simulink library "HardwareIO"  (R2014a)
settings: Solver=ode45  SolverMode=SingleTasking  StartTime=0.0  StopTime=10.0  RelTol=1e-3
values from neighbouring files (symbols this model uses):
  Ts = 0.002    [DSC_Control_Analysis.m]    (also in DSC_Control_Analysis_Exp.m; DSC_Speed_Control_Analysis.m; EC_params_nissan.m; Ext_MPCPara.m = SSD.Ts)
undefined symbols (not defined in the file or in its folder): bit, DiscIntNeverNeededParam, gr, Standard
libraries: canmsglib x6, xpcdiamondlib x2, simulink_extras x2, slrtsoftinglib x2, simulink x1
settings Model: Creator=Shad Laws  LastModifiedBy=cbeal

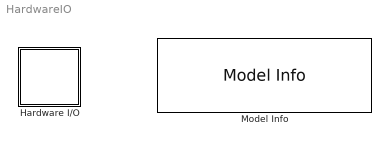
== system HardwareIO ==
  Hardware I/O : Subsystem
      mask init:
      | exist_p1_mdl = sum(strcmp(find_system('p1', 'searchdepth', 0), 'p1'));
      | 
      | if (exist_p1_mdl == 1)
      |     set_param('p1','StopTime','36000');
      |     set_param('p1','StartTime','0');
      | end
      mask Display: disp(['xPC\nI/O']);
  Model Info : simulink/Model-Wide Utilities/Model Info  InitialBlockCM=None  BlockCM=none  Frame=off  DisplayStringWithTags=|  HorizontalTextAlignment=Left  LeftAlignmentValue=0.02  SourceBlockDiagram=HardwareIO  TagMaxNumber=20
      | Last saved on: %<LastModificationDate>
      | Save number: %<ModelVersion>
      | $Revision: 647 $
      | $URL: https://nissan.stanford.edu/nissanxpc/development/HardwareIO.mdl $

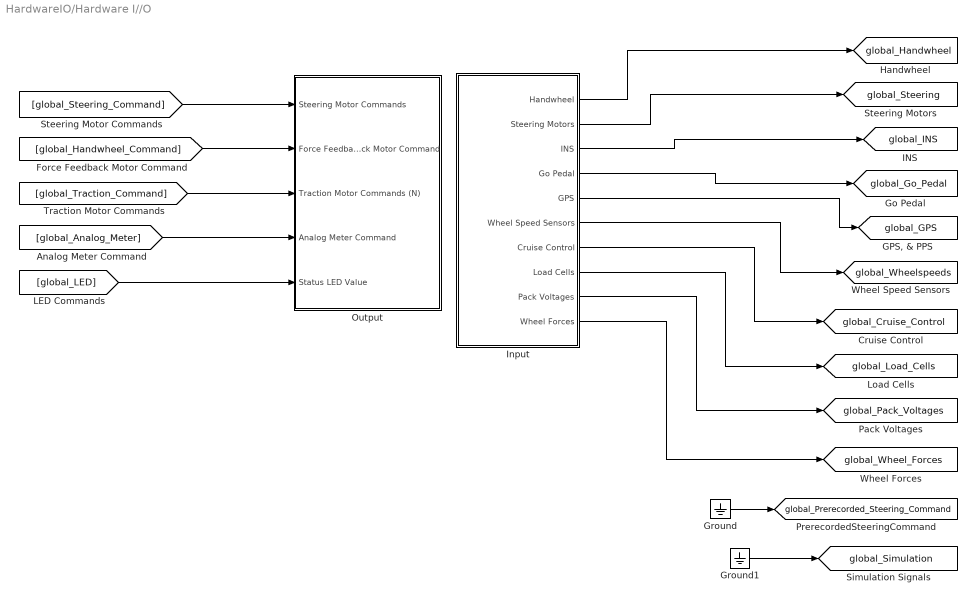
== system HardwareIO/Hardware I//O ==
  Ground : Ground
  Ground1 : Ground
  Input : Subsystem
  Output : Subsystem
  tag scope: global_Cruise_Control=global, global_GPS=global, global_Go_Pedal=global, global_Handwheel=global, global_INS=global, global_Load_Cells=global, global_Pack_Voltages=global, global_Prerecorded_Steering_Command=global, global_Simulation=global, global_Steering=global, global_Wheel_Forces=global, global_Wheelspeeds=global
  wires:
  Input/10(Wheel Forces) -> [global_Wheel_Forces]
  Input/9(Pack Voltages) -> [global_Pack_Voltages]
  Input/8(Load Cells) -> [global_Load_Cells]
  [global_Traction_Command] -> Output/3(Traction Motor Commands (N))
  [global_Analog_Meter] -> Output/4(Analog Meter Command)
  [global_Steering_Command] -> Output/1(Steering Motor Commands)
  [global_Handwheel_Command] -> Output/2(Force Feedback Motor Command)
  [global_LED] -> Output/5(Status LED Value)
  Input/1(Handwheel) -> [global_Handwheel]
  Input/2(Steering Motors) -> [global_Steering]
  Input/3(INS) -> [global_INS]
  Input/4(Go Pedal) -> [global_Go_Pedal]
  Input/5(GPS) -> [global_GPS]
  Input/6(Wheel Speed Sensors) -> [global_Wheelspeeds]
  Input/7(Cruise Control) -> [global_Cruise_Control]
  Ground/1 -> [global_Prerecorded_Steering_Command]
  Ground1/1 -> [global_Simulation]

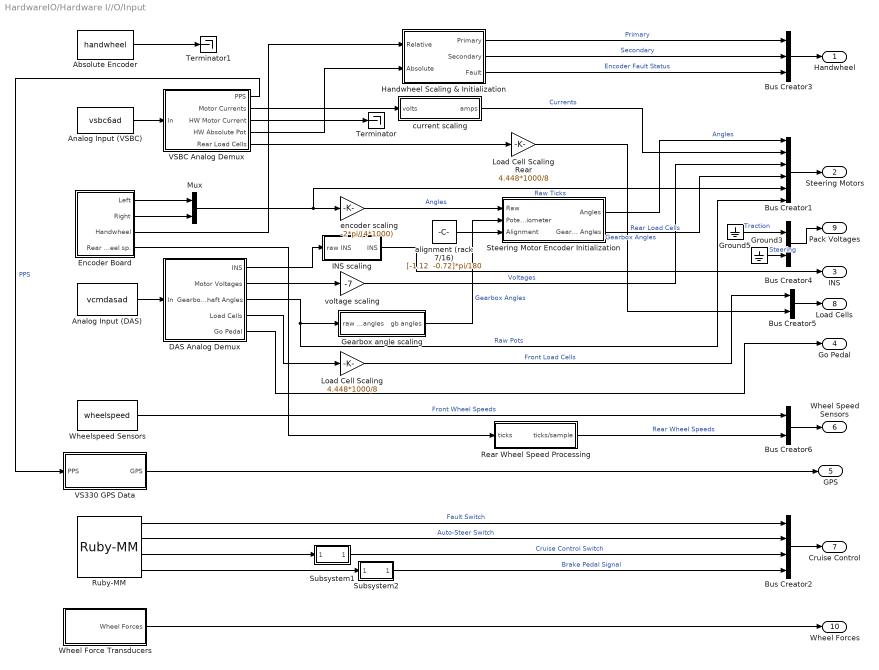
== system HardwareIO/Hardware I//O/Input ==
  Absolute Encoder : S-Function  FunctionName=handwheel  Parameters=Ts  EnableBusSupport=off
  Analog Input (DAS) : S-Function  FunctionName=vcmdasad  Parameters=numChannels, inputVec, sampleTime  EnableBusSupport=off  mask{numChannels=16, inputVec=[4 4 4 4 4 4 4 4 4 4 4 4 4 4 4 4], sampleTime=Ts}
      mask prompts: sampleTime "sample_time"
  Analog Input (VSBC) : S-Function  FunctionName=vsbc6ad  Parameters=numChannels,inpRange,sampTime  EnableBusSupport=off  mask{numChannels=8, inpRange=[4 4 1 4 4 3 3 2], sampTime=Ts}
      mask prompts: numChannels "Number of Channels"; inpRange "Analog Input Range (1: +5; 2: +10; 3: +-5; 4: +-10)"; sampTime "Sampling Time"
  Bus Creator1 : BusCreator  Inputs=6
  Bus Creator2 : BusCreator
  Bus Creator3 : BusCreator  Inputs=3
  Bus Creator4 : BusCreator  Inputs=2
  Bus Creator5 : BusCreator  Inputs=2
  Bus Creator6 : BusCreator  Inputs=2
  DAS Analog Demux : Subsystem
  Encoder Board : Subsystem
  Gearbox angle scaling : Subsystem
  Ground3 : Ground
  Ground5 : Ground
  Handwheel Scaling & Initialization : Subsystem
  INS scaling : Subsystem
  Load Cell Scaling : Gain  Gain=4.448*1000/8  SaturateOnIntegerOverflow=on  OutDataTypeStr=Inherit: Same as input  ParamDataTypeStr=Inherit: Same as input
  Load Cell Scaling Rear : Gain  Gain=4.448*1000/8  SaturateOnIntegerOverflow=on  OutDataTypeStr=Inherit: Same as input  ParamDataTypeStr=Inherit: Same as input
  Mux : Mux  Inputs=2
  Rear Wheel Speed Processing : Subsystem
  Ruby-MM : xpcdiamondlib/Digital Input/Ruby-MM   channel=[5 6 7 8]  port=A  chip=1  sampletime=Ts  baseaddress=0x300
  Steering Motor Encoder Initialization : Subsystem
      mask init:
      | p1_params
  Subsystem1 : Subsystem
      mask Display: disp('!');
  Subsystem2 : Subsystem
      mask Display: disp('!');
  Terminator : Terminator
  Terminator1 : Terminator
  VS330 GPS Data : Subsystem
  VSBC Analog Demux : Subsystem
  Wheel Force Transducers : Subsystem
  Wheelspeed Sensors : S-Function  FunctionName=wheelspeed  Parameters=Ts  EnableBusSupport=off
  alignment (rack 7/16) : Constant  Value="[-1.12  -0.72]*pi/180"
  current scaling : Subsystem
  encoder scaling : Gain  Gain=-2*pi/(4*1000)  SaturateOnIntegerOverflow=on  OutDataTypeStr=Inherit: Same as input  ParamDataTypeStr=Inherit: Same as input
  voltage scaling : Gain  Gain=-7  SaturateOnIntegerOverflow=on  OutDataTypeStr=Inherit: Same as input  ParamDataTypeStr=Inherit: Same as input
  Handwheel : Outport
  Steering Motors : Outport  Port=2
  INS : Outport  Port=3
  Go Pedal : Outport  Port=4
  GPS : Outport  Port=5
  Wheel Speed Sensors : Outport  Port=6
  Cruise Control : Outport  Port=7
  Load Cells : Outport  Port=8
  Pack Voltages : Outport  Port=9
  Wheel Forces : Outport  Port=10
  wires:
  VS330 GPS Data/1(GPS) -> GPS/1
  Wheel Force Transducers/1(Wheel Forces) -> Wheel Forces/1
  Bus Creator6/1 -> Wheel Speed Sensors/1
  Encoder Board/4(Rear wheel sp.) -> Rear Wheel Speed Processing/1(ticks)
  Rear Wheel Speed Processing/1(ticks/sample) -> Bus Creator6/2  "Rear Wheel Speeds"
  Wheelspeed Sensors/1 -> Bus Creator6/1  "Front Wheel Speeds"
  Bus Creator5/1 -> Load Cells/1
  Load Cell Scaling Rear/1 -> Bus Creator5/2  "Rear Load Cells"
  VSBC Analog Demux/5(Rear Load Cells) -> Load Cell Scaling Rear/1
  Load Cell Scaling/1 -> Bus Creator5/1  "Front Load Cells"
  Absolute Encoder/1 -> Terminator1/1
  VSBC Analog Demux/3(HW Motor Current) -> Terminator/1
  Encoder Board/3(Handwheel) -> Handwheel Scaling & Initialization/1(Relative)
  Ground3/1 -> Bus Creator4/2  "Steering"
  Bus Creator4/1 -> Pack Voltages/1
  DAS Analog Demux/4(Load Cells) -> Load Cell Scaling/1
  Handwheel Scaling & Initialization/2(Secondary) -> Bus Creator3/2  "Secondary"
  Bus Creator3/1 -> Handwheel/1
  DAS Analog Demux/5(Go Pedal) -> Go Pedal/1
  Bus Creator2/1 -> Cruise Control/1
  DAS Analog Demux/2(Motor Voltages) -> voltage scaling/1
  voltage scaling/1 -> Bus Creator1/3  "Voltages"
  Mux/1 -> encoder scaling/1, Bus Creator1/5  "Raw Ticks"
  Encoder Board/2(Right) -> Mux/2
  Encoder Board/1(Left) -> Mux/1
  Analog Input (VSBC)/1 -> VSBC Analog Demux/1(In)
  VSBC Analog Demux/1(PPS) -> VS330 GPS Data/1(PPS)  "PPS"
  Bus Creator1/1 -> Steering Motors/1
  VSBC Analog Demux/2(Motor Currents) -> current scaling/1(volts)
  current scaling/1(amps) -> Bus Creator1/2  "Currents"
  INS scaling/1(INS) -> INS/1
  DAS Analog Demux/1(INS) -> INS scaling/1(raw INS)
  Analog Input (DAS)/1 -> DAS Analog Demux/1(In)
  DAS Analog Demux/3(Gearbox Shaft Angles) -> Bus Creator1/6, Gearbox angle scaling/1(raw gb angles)  "Raw Pots"
  Gearbox angle scaling/1(gb angles) -> Steering Motor Encoder Initialization/2(Potentiometer)  "Gearbox Angles"
  Subsystem1/1(Out1) -> Bus Creator2/3  "Cruise Control Switch"
  Subsystem2/1(Out1) -> Bus Creator2/4  "Brake Pedal Signal"
  encoder scaling/1 -> Steering Motor Encoder Initialization/1(Raw)  "Angles"
  Handwheel Scaling & Initialization/3(Fault) -> Bus Creator3/3  "Encoder Fault Status"
  Steering Motor Encoder Initialization/1(Angles) -> Bus Creator1/1  "Angles"
  alignment (rack 7/16)/1 -> Steering Motor Encoder Initialization/3(Alignment)
  Steering Motor Encoder Initialization/2(Gearbox Angles) -> Bus Creator1/4  "Gearbox Angles"
  Ruby-MM/3 -> Subsystem1/1(In1)
  Ruby-MM/4 -> Subsystem2/1(In1)
  Ruby-MM/2 -> Bus Creator2/2  "Auto-Steer Switch"
  Ruby-MM/1 -> Bus Creator2/1  "Fault Switch"
  Ground5/1 -> Bus Creator4/1  "Traction"
  Handwheel Scaling & Initialization/1(Primary) -> Bus Creator3/1  "Primary"
  VSBC Analog Demux/4(HW Absolute Pot) -> Handwheel Scaling & Initialization/2(Absolute)

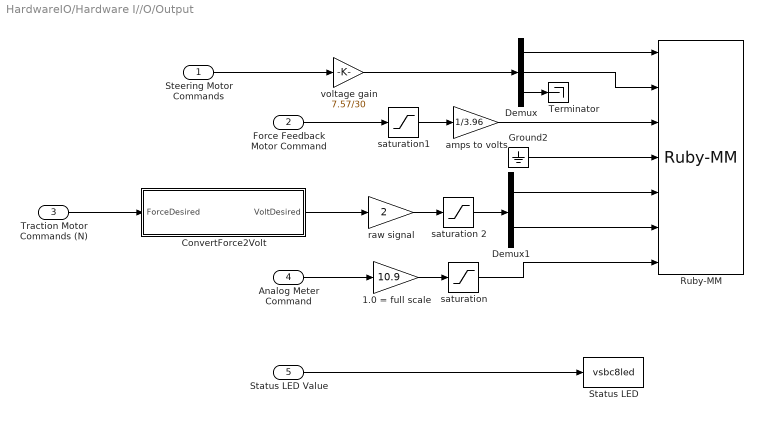
== system HardwareIO/Hardware I//O/Output ==
  Steering Motor Commands : Inport
  Force Feedback Motor Command : Inport  Port=2
  Traction Motor Commands (N) : Inport  Port=3
  Analog Meter Command : Inport  Port=4
  Status LED Value : Inport  Port=5
  1.0 = full scale : Gain  Gain=10.9  SaturateOnIntegerOverflow=on  OutDataTypeStr=Inherit: Same as input  ParamDataTypeStr=Inherit: Same as input
  ConvertForce2Volt : Subsystem  TreatAsAtomicUnit=on
  Demux : Demux  Outputs=[1 1 -1]
  Demux1 : Demux  Outputs=2
  Ground2 : Ground
  "Ruby-MM " : xpcdiamondlib/D//A/Ruby-MM   channel=[1 2 3 4 5 6 7]  range0=+-10  range1=+-10  reset=[1 1 1 1 1 1 1]  initValue=[0 0 0 0 0 0 0]  st=Ts  baseaddress=0x300
  Status LED : S-Function  FunctionName=vsbc8led  EnableBusSupport=off
  Terminator : Terminator
  amps to volts : Gain  Gain=1/3.96  SaturateOnIntegerOverflow=on  OutDataTypeStr=Inherit: Same as input  ParamDataTypeStr=Inherit: Same as input
  raw signal : Gain  Gain=2  SaturateOnIntegerOverflow=on  OutDataTypeStr=Inherit: Same as input  ParamDataTypeStr=Inherit: Same as input
  saturation : Saturate  UpperLimit=11  LowerLimit=0
  saturation 2 : Saturate  UpperLimit=6  LowerLimit=0  OutDataTypeStr=Inherit: Inherit via back propagation
  saturation1 : Saturate  UpperLimit=2  LowerLimit=-2
  voltage gain : Gain  Gain=7.57/30  SaturateOnIntegerOverflow=on  OutDataTypeStr=Inherit: Same as input  ParamDataTypeStr=Inherit: Same as input
  wires:
  Demux/3 -> Terminator/1
  ConvertForce2Volt/1(VoltDesired) -> raw signal/1
  amps to volts/1 -> "Ruby-MM "/3
  Force Feedback Motor Command/1 -> saturation1/1
  raw signal/1 -> saturation 2/1
  saturation 2/1 -> Demux1/1
  saturation/1 -> "Ruby-MM "/7
  Demux1/2 -> "Ruby-MM "/6
  Steering Motor Commands/1 -> voltage gain/1
  voltage gain/1 -> Demux/1
  1.0 = full scale/1 -> saturation/1
  Ground2/1 -> "Ruby-MM "/4
  Demux/2 -> "Ruby-MM "/2
  Demux/1 -> "Ruby-MM "/1
  Status LED Value/1 -> Status LED/1
  Demux1/1 -> "Ruby-MM "/5
  Traction Motor Commands (N)/1 -> ConvertForce2Volt/1(ForceDesired)
  Analog Meter Command/1 -> 1.0 = full scale/1
  saturation1/1 -> amps to volts/1

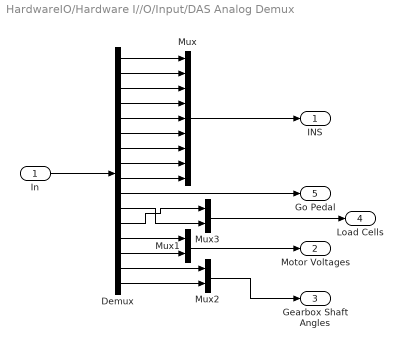
== system HardwareIO/Hardware I//O/Input/DAS Analog Demux ==
  In : Inport
  Demux : Demux  Outputs=16
  Mux : Mux  Inputs=9
  Mux1 : Mux  Inputs=2
  Mux2 : Mux  Inputs=2
  Mux3 : Mux  Inputs=2
  INS : Outport
  Motor Voltages : Outport  Port=2
  Gearbox Shaft Angles : Outport  Port=3
  Load Cells : Outport  Port=4
  Go Pedal : Outport  Port=5
  wires:
  Demux/10 -> Go Pedal/1
  Mux3/1 -> Load Cells/1
  Demux/16 -> Mux2/2
  Demux/15 -> Mux2/1
  Demux/2 -> Mux/2
  Demux/14 -> Mux1/2
  Demux/13 -> Mux1/1
  Mux1/1 -> Motor Voltages/1
  Mux/1 -> INS/1
  Demux/9 -> Mux/9
  Demux/8 -> Mux/8
  Demux/7 -> Mux/7
  Demux/6 -> Mux/6
  Demux/5 -> Mux/5
  Demux/4 -> Mux/4
  Demux/3 -> Mux/3
  Demux/1 -> Mux/1
  In/1 -> Demux/1
  Mux2/1 -> Gearbox Shaft Angles/1
  Demux/11 -> Mux3/2
  Demux/12 -> Mux3/1

== system HardwareIO/Hardware I//O/Input/Encoder Board ==
  Mux : Mux  Inputs=2
  "encoder board " : S-Function  FunctionName=UltimateEncoder  Parameters=TSamp,NC,BA,[R1 R2 R3 R4 R5 R6 ]  EnableBusSupport=off  mask{TSamp=Ts, BA=528, NC=5, R1=on, R2=on, R3=on, R4=off, R5=off, R6=off}
      mask prompts: TSamp "Sampling Rate"; BA "Base Adress (Base 10)"; NC "Number of Channels"; R1 "Unwrap Channel 1"; R2 "Unwrap Channel 2"; R3 "Unwrap Channel 3"; R4 "Unwrap Channel 4"; R5 "Unwrap Channel 5"; R6 "Unwrap Channel 6"
  reset : Constant  Value=[1 1 1 0 0]
  Left : Outport
  Right : Outport  Port=2
  Handwheel : Outport  Port=3
  Rear wheel sp. : Outport  Port=4
  wires:
  Mux/1 -> Rear wheel sp./1
  "encoder board "/5 -> Mux/2
  "encoder board "/4 -> Mux/1
  "encoder board "/3 -> Handwheel/1
  reset/1 -> "encoder board "/1
  "encoder board "/1 -> Left/1
  "encoder board "/2 -> Right/1

== system HardwareIO/Hardware I//O/Input/Gearbox angle scaling ==
  raw gb angles : Inport
  Pot readings with wheels centered : Constant  Value=[ -2.041; -1.733 ]
  Sum : Sum  Inputs=|++  SaturateOnIntegerOverflow=on
  Volts/Rad (Left/right pots wired in reverse) : Gain  Gain=[1/ -1.31; 1/1.254]  SaturateOnIntegerOverflow=on  OutDataTypeStr=Inherit: Same as input  ParamDataTypeStr=Inherit: Same as input
  gb angles : Outport
  wires:
  Sum/1 -> Volts/Rad (Left/right pots wired in reverse)/1
  raw gb angles/1 -> Sum/1
  Pot readings with wheels centered/1 -> Sum/2
  Volts/Rad (Left/right pots wired in reverse)/1 -> gb angles/1

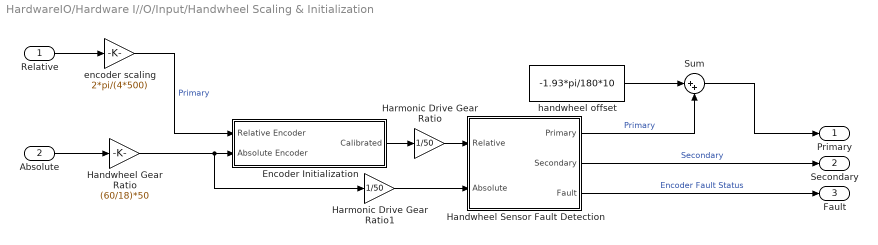
== system HardwareIO/Hardware I//O/Input/Handwheel Scaling & Initialization ==
  Relative : Inport
  Absolute : Inport  Port=2
  Encoder Initialization : Subsystem
  Handwheel Gear Ratio : Gain  Gain=(60/18)*50  SaturateOnIntegerOverflow=on  OutDataTypeStr=Inherit: Same as input  ParamDataTypeStr=Inherit: Same as input
  Handwheel Sensor Fault Detection : Subsystem
  Harmonic Drive Gear Ratio : Gain  Gain=1/50  SaturateOnIntegerOverflow=on  OutDataTypeStr=Inherit: Same as input  ParamDataTypeStr=Inherit: Same as input
  Harmonic Drive Gear Ratio1 : Gain  Gain=1/50  SaturateOnIntegerOverflow=on  OutDataTypeStr=Inherit: Same as input  ParamDataTypeStr=Inherit: Same as input
  Sum : Sum  Inputs=|++
  encoder scaling : Gain  Gain=2*pi/(4*500)  SaturateOnIntegerOverflow=on  OutDataTypeStr=Inherit: Same as input  ParamDataTypeStr=Inherit: Same as input
  handwheel offset : Constant  Value=-1.93*pi/180*10
  Primary : Outport
  Secondary : Outport  Port=2
  Fault : Outport  Port=3
  wires:
  Handwheel Sensor Fault Detection/1(Primary) -> Sum/2  "Primary"
  Sum/1 -> Primary/1
  handwheel offset/1 -> Sum/1
  Harmonic Drive Gear Ratio1/1 -> Handwheel Sensor Fault Detection/2(Absolute)
  Absolute/1 -> Handwheel Gear Ratio/1
  Relative/1 -> encoder scaling/1
  Harmonic Drive Gear Ratio/1 -> Handwheel Sensor Fault Detection/1(Relative)
  Handwheel Sensor Fault Detection/2(Secondary) -> Secondary/1  "Secondary"
  Encoder Initialization/1(Calibrated) -> Harmonic Drive Gear Ratio/1
  Handwheel Sensor Fault Detection/3(Fault) -> Fault/1  "Encoder Fault Status"
  Handwheel Gear Ratio/1 -> Harmonic Drive Gear Ratio1/1, Encoder Initialization/2(Absolute Encoder)
  encoder scaling/1 -> Encoder Initialization/1(Relative Encoder)  "Primary"

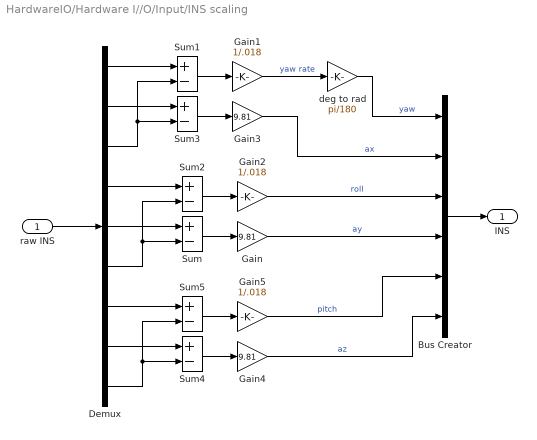
== system HardwareIO/Hardware I//O/Input/INS scaling ==
  raw INS : Inport
  Bus Creator : BusCreator  Inputs=6
  Demux : Demux  Outputs=9
  Gain : Gain  Gain=9.81  SaturateOnIntegerOverflow=on  OutDataTypeStr=Inherit: Same as input  ParamDataTypeStr=Inherit: Same as input
  Gain1 : Gain  Gain=1/.018  SaturateOnIntegerOverflow=on  OutDataTypeStr=Inherit: Same as input  ParamDataTypeStr=Inherit: Same as input
  Gain2 : Gain  Gain=1/.018  SaturateOnIntegerOverflow=on  OutDataTypeStr=Inherit: Same as input  ParamDataTypeStr=Inherit: Same as input
  Gain3 : Gain  Gain=9.81  SaturateOnIntegerOverflow=on  OutDataTypeStr=Inherit: Same as input  ParamDataTypeStr=Inherit: Same as input
  Gain4 : Gain  Gain=9.81  SaturateOnIntegerOverflow=on  OutDataTypeStr=Inherit: Same as input  ParamDataTypeStr=Inherit: Same as input
  Gain5 : Gain  Gain=1/.018  SaturateOnIntegerOverflow=on  OutDataTypeStr=Inherit: Same as input  ParamDataTypeStr=Inherit: Same as input
  Sum{,1..5} (6 alike) : Sum  Inputs=+-  SaturateOnIntegerOverflow=on  InputSameDT=on  OutDataTypeStr=Inherit: Same as first input
  deg to rad : Gain  Gain=pi/180  SaturateOnIntegerOverflow=on  OutDataTypeStr=Inherit: Same as input  ParamDataTypeStr=Inherit: Same as input
  INS : Outport
  wires:
  Bus Creator/1 -> INS/1
  deg to rad/1 -> Bus Creator/1  "yaw"
  Demux/9 -> Sum4/2, Sum5/2
  Demux/5 -> Sum/1
  Demux/8 -> Sum4/1
  Demux/7 -> Sum5/1
  Sum4/1 -> Gain4/1
  Sum5/1 -> Gain5/1
  Gain4/1 -> Bus Creator/6  "az"
  Gain5/1 -> Bus Creator/5  "pitch"
  raw INS/1 -> Demux/1
  Sum/1 -> Gain/1
  Sum1/1 -> Gain1/1
  Sum2/1 -> Gain2/1
  Sum3/1 -> Gain3/1
  Gain/1 -> Bus Creator/4  "ay"
  Gain1/1 -> deg to rad/1  "yaw rate"
  Gain2/1 -> Bus Creator/3  "roll"
  Gain3/1 -> Bus Creator/2  "ax"
  Demux/1 -> Sum1/1
  Demux/3 -> Sum1/2, Sum3/2
  Demux/2 -> Sum3/1
  Demux/4 -> Sum2/1
  Demux/6 -> Sum/2, Sum2/2

== system HardwareIO/Hardware I//O/Input/Rear Wheel Speed Processing ==
  ticks : Inport
  Demux : Demux  Outputs=2
  Mux : Mux  Inputs=2
  Speed Calc : Subsystem  mask{range=65536}
      mask prompts: range "Wrap range"
      mask Display: disp(range);
  Speed Calc1 : Subsystem  mask{range=65536}
      mask prompts: range "Wrap range"
      mask Display: disp(range);
  de-quadrature : Gain  Gain=1/2
  ticks/sample : Outport
  wires:
  de-quadrature/1 -> ticks/sample/1
  Mux/1 -> de-quadrature/1
  Speed Calc1/1(Speed) -> Mux/2
  Demux/2 -> Speed Calc1/1(Distance)
  Speed Calc/1(Speed) -> Mux/1
  Demux/1 -> Speed Calc/1(Distance)
  ticks/1 -> Demux/1

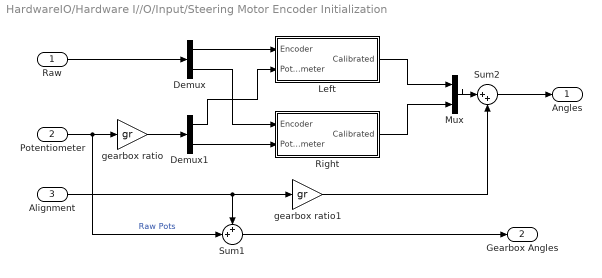
== system HardwareIO/Hardware I//O/Input/Steering Motor Encoder Initialization ==
  Raw : Inport
  Potentiometer : Inport  Port=2
  Alignment : Inport  Port=3
  Demux : Demux  Outputs=2
  Demux1 : Demux  Outputs=2
  Left : Subsystem
  Mux : Mux  Inputs=2
  Right : Subsystem
  Sum1 : Sum  Inputs=++|
  Sum2 : Sum  Inputs=|++
  gearbox ratio : Gain  Gain=gr  SaturateOnIntegerOverflow=on  OutDataTypeStr=Inherit: Same as input  ParamDataTypeStr=Inherit: Same as input
  gearbox ratio1 : Gain  Gain=gr  SaturateOnIntegerOverflow=on  OutDataTypeStr=Inherit: Same as input  ParamDataTypeStr=Inherit: Same as input
  Angles : Outport
  Gearbox Angles : Outport  Port=2
  wires:
  Demux1/2 -> Right/2(Potentiometer)
  Demux1/1 -> Left/2(Potentiometer)
  Demux/2 -> Right/1(Encoder)
  Demux/1 -> Left/1(Encoder)
  Left/1(Calibrated) -> Mux/1
  Potentiometer/1 -> gearbox ratio/1, Sum1/2  "Raw Pots"
  Raw/1 -> Demux/1
  gearbox ratio/1 -> Demux1/1
  Right/1(Calibrated) -> Mux/2
  Mux/1 -> Sum2/1
  Sum2/1 -> Angles/1
  Alignment/1 -> gearbox ratio1/1, Sum1/1
  gearbox ratio1/1 -> Sum2/2
  Sum1/1 -> Gearbox Angles/1

== system HardwareIO/Hardware I//O/Input/Subsystem1 ==
  In1 : Inport
  Constant : Constant
  Sum : Sum  Inputs=+-|
  Out1 : Outport
  wires:
  Constant/1 -> Sum/1
  In1/1 -> Sum/2
  Sum/1 -> Out1/1

== system HardwareIO/Hardware I//O/Input/Subsystem2 ==
  In1 : Inport
  Constant : Constant
  Sum : Sum  Inputs=+-|
  Out1 : Outport
  wires:
  Sum/1 -> Out1/1
  In1/1 -> Sum/2
  Constant/1 -> Sum/1

== system HardwareIO/Hardware I//O/Input/VS330 GPS Data ==
  note: Do not reorder the signals in
      | GPS or DataDescription will
      | not match the data.
  PPS : Inport
  Bus Creator : BusCreator  Inputs=28
  Demux : Demux  Outputs=24
  Hemisphere VS330 : S-Function  FunctionName=vs330_bin3_rcv  Parameters=Ts  EnableBusSupport=off
  Roll Axis Reversed : Gain  Gain=-1
  Subsystem : Subsystem
  Terminator2 : Terminator
  GPS : Outport
  wires:
  Roll Axis Reversed/1 -> Bus Creator/14  "Roll Angle"
  Demux/12 -> Roll Axis Reversed/1  "Roll Angle"
  Subsystem/3(Z) -> Bus Creator/9  "ECEF Z"
  Subsystem/2(Y) -> Bus Creator/8  "ECEF Y"
  Subsystem/1(X) -> Bus Creator/7  "ECEF X"
  Demux/7 -> Bus Creator/6, Subsystem/3(Alt)  "Altitude"
  Demux/6 -> Bus Creator/5, Subsystem/2(Long)  "Longitude"
  Demux/5 -> Bus Creator/4, Subsystem/1(Lat)  "Latitude"
  Demux/18 -> Bus Creator/22  "Vert RMS"
  Demux/23 -> Bus Creator/27  "Cov EU"
  Demux/14 -> Bus Creator/16  "Attitude Status"
  Demux/15 -> Bus Creator/19  "Yaw stddev"
  Demux/21 -> Bus Creator/25  "Cov NU"
  Demux/1 -> Bus Creator/2  "ToW"
  Demux/17 -> Bus Creator/21  "Hor RMS"
  Demux/4 -> Bus Creator/15  "Nav Mode"
  Demux/3 -> Bus Creator/17  "Sats Used"
  Demux/22 -> Bus Creator/26  "Cov EE"
  Demux/20 -> Bus Creator/24  "Cov NE"
  Demux/24 -> Bus Creator/28  "Cov UU"
  Demux/11 -> Bus Creator/13  "Heading"
  Demux/2 -> Bus Creator/3  "Wk Num"
  Demux/19 -> Bus Creator/23  "Cov NN"
  Demux/9 -> Bus Creator/11  "Vert Vel"
  Demux/8 -> Bus Creator/10  "Hor Speed"
  Demux/10 -> Bus Creator/12  "CoG"
  Demux/13 -> Bus Creator/18  "Diff Age"
  Demux/16 -> Bus Creator/20  "Roll stddev"
  Hemisphere VS330/1 -> Demux/1
  Hemisphere VS330/2 -> Terminator2/1
  Bus Creator/1 -> GPS/1
  PPS/1 -> Bus Creator/1

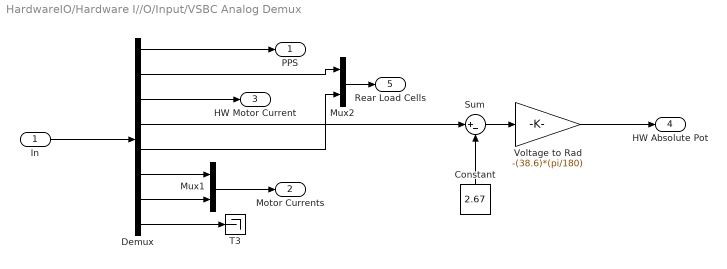
== system HardwareIO/Hardware I//O/Input/VSBC Analog Demux ==
  In : Inport
  Constant : Constant  Value=2.67
  Demux : Demux  Outputs=8
  Mux1 : Mux  Inputs=2
  Mux2 : Mux  Inputs=2
  Sum : Sum  Inputs=|+-
  T3 : Terminator
  Voltage to Rad : Gain  Gain=-(38.6)*(pi/180)
  PPS : Outport
  Motor Currents : Outport  Port=2
  HW Motor Current : Outport  Port=3
  HW Absolute Pot : Outport  Port=4
  Rear Load Cells : Outport  Port=5
  wires:
  Mux2/1 -> Rear Load Cells/1
  Demux/5 -> Mux2/2
  Demux/2 -> Mux2/1
  Constant/1 -> Sum/2
  Sum/1 -> Voltage to Rad/1
  Demux/4 -> Sum/1
  Voltage to Rad/1 -> HW Absolute Pot/1
  Demux/8 -> T3/1
  Demux/1 -> PPS/1
  Demux/3 -> HW Motor Current/1
  Demux/6 -> Mux1/1
  Demux/7 -> Mux1/2
  In/1 -> Demux/1
  Mux1/1 -> Motor Currents/1

== system HardwareIO/Hardware I//O/Input/Wheel Force Transducers ==
  Bus Creator : BusCreator  Inputs=20
  CAN Unpack : canmsglib/CAN Unpack  MsgList=(none)  MsgName=CAN Msg  MsgIDType=Standard (11-bit identifier)  MsgIdentifier=460  MsgLength=8  SignalInfo=LF_X_Force$0$16$1$1$1$0$1.220703125$0$-Inf$Inf$#LF_Y_Force$16$16$1$1$1$0$0.6103515625$0$-Inf$Inf$#LF_Z_Force$32$16$1$1$1$0$1.220703125$0$-Inf$Inf$#LF_MX_Moment$48$16$1$1$1$0$0.18310546875$0$-Inf$Inf$#  NSignals=4  IDPort=off  TimestampPort=off  ErrorPort=off  RemotePort=off  LengthPort=off  StatusPort=on  StartBits=str2num('[int32(0);int32(16);int32(32);int32(48)]')  SignalSizes=str2num('[int32(16);int32(16);int32(16);int32(16)]')  ByteOrders=str2num('[int32(1);int32(1);int32(1);int32(1)]')  DataTypes=str2num('[int32(1);int32(1);int32(1);int32(1)]')  MultiplexTypes=str2num('[int32(1);int32(1);int32(1);int32(1)]')  MultiplexValues=str2num('[double(0);double(0);double(0);double(0)]')  Factors=str2num('[double(1.220703125);double(0.6103515625);double(1.220703125);double(0.18310546875)]')  Offsets=str2num('[double(0);double(0);double(0);double(0)]')  Minimums=str2num('[double(-Inf);double(-Inf);double(-Inf);double(-Inf)]')  Maximums=str2num('[double(Inf);double(Inf);double(Inf);double(Inf)]')
  CAN Unpack1 : canmsglib/CAN Unpack  MsgList=(none)  MsgName=CAN Msg  MsgIDType=Standard (11-bit identifier)  MsgIdentifier=1484  MsgLength=8  SignalInfo=LF_MY_Moment$0$16$1$1$1$0$0.18310546875$0$-Inf$Inf$#LF_MZ_Moment$16$16$1$1$1$0$0.18310546875$0$-Inf$Inf$#LF_Velocity$32$16$1$1$1$0$0.06103515625$0$-Inf$Inf$#LF_Position$48$16$1$1$1$0$0.010986328125$0$-Inf$Inf$#  NSignals=4  IDPort=off  TimestampPort=off  ErrorPort=off  RemotePort=off  LengthPort=off  StatusPort=on  StartBits=str2num('[int32(0);int32(16);int32(32);int32(48)]')  SignalSizes=str2num('[int32(16);int32(16);int32(16);int32(16)]')  ByteOrders=str2num('[int32(1);int32(1);int32(1);int32(1)]')  DataTypes=str2num('[int32(1);int32(1);int32(1);int32(1)]')  MultiplexTypes=str2num('[int32(1);int32(1);int32(1);int32(1)]')  MultiplexValues=str2num('[double(0);double(0);double(0);double(0)]')  Factors=str2num('[double(0.18310546875);double(0.18310546875);double(0.06103515625);double(0.010986328125)]')  Offsets=str2num('[double(0);double(0);double(0);double(0)]')  Minimums=str2num('[double(-Inf);double(-Inf);double(-Inf);double(-Inf)]')  Maximums=str2num('[double(Inf);double(Inf);double(Inf);double(Inf)]')
  CAN Unpack2 : canmsglib/CAN Unpack  MsgList=(none)  MsgName=CAN Msg  MsgIDType=Standard (11-bit identifier)  MsgIdentifier=972  MsgLength=8  SignalInfo=LF_X_Accel$0$16$1$1$1$0$0.0030517578125$0$-Inf$Inf$#LF_Y_Accel$16$16$1$1$1$0$0.0030517578125$0$-Inf$Inf$#  NSignals=2  IDPort=off  TimestampPort=off  ErrorPort=off  RemotePort=off  LengthPort=off  StatusPort=on  StartBits=str2num('[int32(0);int32(16)]')  SignalSizes=str2num('[int32(16);int32(16)]')  ByteOrders=str2num('[int32(1);int32(1)]')  DataTypes=str2num('[int32(1);int32(1)]')  MultiplexTypes=str2num('[int32(1);int32(1)]')  MultiplexValues=str2num('[double(0);double(0)]')  Factors=str2num('[double(0.0030517578125);double(0.0030517578125)]')  Offsets=str2num('[double(0);double(0)]')  Minimums=str2num('[double(-Inf);double(-Inf)]')  Maximums=str2num('[double(Inf);double(Inf)]')
  CAN Unpack3 : canmsglib/CAN Unpack  MsgList=(none)  MsgName=CAN Msg  MsgIDType=Standard (11-bit identifier)  MsgIdentifier=455  MsgLength=8  SignalInfo=RF_X_Force$0$16$1$1$1$0$1.220703125$0$-Inf$Inf$#RF_Y_Force$16$16$1$1$1$0$0.6103515625$0$-Inf$Inf$#RF_Z_Force$32$16$1$1$1$0$1.220703125$0$-Inf$Inf$#RF_MX_Moment$48$16$1$1$1$0$0.18310546875$0$-Inf$Inf$#  NSignals=4  IDPort=off  TimestampPort=off  ErrorPort=off  RemotePort=off  LengthPort=off  StatusPort=on  StartBits=str2num('[int32(0);int32(16);int32(32);int32(48)]')  SignalSizes=str2num('[int32(16);int32(16);int32(16);int32(16)]')  ByteOrders=str2num('[int32(1);int32(1);int32(1);int32(1)]')  DataTypes=str2num('[int32(1);int32(1);int32(1);int32(1)]')  MultiplexTypes=str2num('[int32(1);int32(1);int32(1);int32(1)]')  MultiplexValues=str2num('[double(0);double(0);double(0);double(0)]')  Factors=str2num('[double(1.220703125);double(0.6103515625);double(1.220703125);double(0.18310546875)]')  Offsets=str2num('[double(0);double(0);double(0);double(0)]')  Minimums=str2num('[double(-Inf);double(-Inf);double(-Inf);double(-Inf)]')  Maximums=str2num('[double(Inf);double(Inf);double(Inf);double(Inf)]')
  CAN Unpack4 : canmsglib/CAN Unpack  MsgList=(none)  MsgName=CAN Msg  MsgIDType=Standard (11-bit identifier)  MsgIdentifier=1479  MsgLength=8  SignalInfo=RF_MY_Moment$0$16$1$1$1$0$0.18310546875$0$-Inf$Inf$#RF_MZ_Moment$16$16$1$1$1$0$0.18310546875$0$-Inf$Inf$#RF_Velocity$32$16$1$1$1$0$0.06103515625$0$-Inf$Inf$#RF_Position$48$16$1$1$1$0$0.010986328125$0$-Inf$Inf$#  NSignals=4  IDPort=off  TimestampPort=off  ErrorPort=off  RemotePort=off  LengthPort=off  StatusPort=on  StartBits=str2num('[int32(0);int32(16);int32(32);int32(48)]')  SignalSizes=str2num('[int32(16);int32(16);int32(16);int32(16)]')  ByteOrders=str2num('[int32(1);int32(1);int32(1);int32(1)]')  DataTypes=str2num('[int32(1);int32(1);int32(1);int32(1)]')  MultiplexTypes=str2num('[int32(1);int32(1);int32(1);int32(1)]')  MultiplexValues=str2num('[double(0);double(0);double(0);double(0)]')  Factors=str2num('[double(0.18310546875);double(0.18310546875);double(0.06103515625);double(0.010986328125)]')  Offsets=str2num('[double(0);double(0);double(0);double(0)]')  Minimums=str2num('[double(-Inf);double(-Inf);double(-Inf);double(-Inf)]')  Maximums=str2num('[double(Inf);double(Inf);double(Inf);double(Inf)]')
  CAN Unpack5 : canmsglib/CAN Unpack  MsgList=(none)  MsgName=CAN Msg  MsgIDType=Standard (11-bit identifier)  MsgIdentifier=967  MsgLength=8  SignalInfo=RF_X_Accel$0$16$1$1$1$0$0.0030517578125$0$-Inf$Inf$#RF_Y_Accel$16$16$1$1$1$0$0.0030517578125$0$-Inf$Inf$#  NSignals=2  IDPort=off  TimestampPort=off  ErrorPort=off  RemotePort=off  LengthPort=off  StatusPort=on  StartBits=str2num('[int32(0);int32(16)]')  SignalSizes=str2num('[int32(16);int32(16)]')  ByteOrders=str2num('[int32(1);int32(1)]')  DataTypes=str2num('[int32(1);int32(1)]')  MultiplexTypes=str2num('[int32(1);int32(1)]')  MultiplexValues=str2num('[double(0);double(0)]')  Factors=str2num('[double(0.0030517578125);double(0.0030517578125)]')  Offsets=str2num('[double(0);double(0)]')  Minimums=str2num('[double(-Inf);double(-Inf)]')  Maximums=str2num('[double(Inf);double(Inf)]')
  "Receive " : slrtsoftinglib/CAN-AC2-104 SJA 1000/Receive   board=1  canPort=CAN 1  range=Standard (11-bit)  ids=[460,455,1484,1479,972,967]  lengths=[8,8,8,8,8,8]  output=CAN_MESSAGE data type  inten=off  ts=-1  ididx=[1,0,5,4,3,2]
  "Setup " : slrtsoftinglib/CAN-AC2-104 SJA 1000/Setup   board=1  can1Baudrate=1 MBaud  can1UserBR=[1,1,4,3]  can2Baudrate=1 MBaud  can2UserBR=[1,1,4,3]  init=[]  term=[]  bus_off_out=off  bus_off_rec=Off  ioBaseAddressL=0x28C  memBaseAddressL=0xd0000  intNo=None
  Wheel Forces : Outport
  wires:
  "Receive "/6 -> CAN Unpack5/1
  "Receive "/4 -> CAN Unpack4/1
  "Receive "/2 -> CAN Unpack3/1
  "Receive "/3 -> CAN Unpack1/1
  "Receive "/1 -> CAN Unpack/1
  "Receive "/5 -> CAN Unpack2/1
  CAN Unpack1/2 -> Bus Creator/11  "LF_Mz"
  CAN Unpack5/2 -> Bus Creator/20  "RF_ay"
  CAN Unpack5/1 -> Bus Creator/18  "RF_ax"
  CAN Unpack4/4 -> Bus Creator/16  "RF_theta"
  CAN Unpack4/3 -> Bus Creator/14  "RF_omega"
  CAN Unpack4/2 -> Bus Creator/12  "RF_Mz"
  CAN Unpack4/1 -> Bus Creator/10  "RF_My"
  CAN Unpack3/4 -> Bus Creator/8  "RF_Mx"
  CAN Unpack3/3 -> Bus Creator/6  "RF_Fz"
  CAN Unpack3/2 -> Bus Creator/4  "RF_Fy"
  CAN Unpack3/1 -> Bus Creator/2  "RF_Fx"
  CAN Unpack2/2 -> Bus Creator/19  "LF_ay"
  CAN Unpack2/1 -> Bus Creator/17  "LF_ax"
  CAN Unpack1/4 -> Bus Creator/15  "LF_theta"
  CAN Unpack1/3 -> Bus Creator/13  "LF_omega"
  CAN Unpack1/1 -> Bus Creator/9  "LF_My"
  Bus Creator/1 -> Wheel Forces/1
  CAN Unpack/4 -> Bus Creator/7  "LF_Mx"
  CAN Unpack/3 -> Bus Creator/5  "LF_Fz"
  CAN Unpack/2 -> Bus Creator/3  "LF_Fy"
  CAN Unpack/1 -> Bus Creator/1  "LF_Fx"

== system HardwareIO/Hardware I//O/Input/current scaling ==
  volts : Inport
  Constant : Constant  Value=-5.39
  Sum : Sum  Inputs=|++  SaturateOnIntegerOverflow=on
  current scaling : Gain  Gain=30/7.5*3.3  SaturateOnIntegerOverflow=on  OutDataTypeStr=Inherit: Same as input  ParamDataTypeStr=Inherit: Same as input
  amps : Outport
  wires:
  Constant/1 -> Sum/2
  Sum/1 -> amps/1
  current scaling/1 -> Sum/1
  volts/1 -> current scaling/1

== system HardwareIO/Hardware I//O/Output/ConvertForce2Volt ==
  ForceDesired : Inport
  VoltDesired : Outport
  wires:
  ForceDesired/1 -> VoltDesired/1

== system HardwareIO/Hardware I//O/Input/Handwheel Scaling & Initialization/Encoder Initialization ==
  Relative Encoder : Inport
  Absolute Encoder : Inport  Port=2
  Encoder Initializer : S-Function  FunctionName=encoderinit  Parameters=sampleTime,firstDelay,secondDelay  EnableBusSupport=off  mask{sampleTime=Ts, firstDelay=.1, secondDelay=.2}
      mask prompts: sampleTime "Sample time"; firstDelay "First calibration time"; secondDelay "Second calibration time"
      mask Display:
      | port_label('input',1,'Unwrapped');
      | port_label('input',2,'Raw');
      | port_label('input',3,'Absolute');
      | port_label('output',1,'Calibrated');
  Unwrapper : S-Function  FunctionName=unwrapper  Parameters=Ts,2*pi  EnableBusSupport=off
      mask Display: disp('2*pi')
  Calibrated : Outport
  wires:
  Encoder Initializer/1 -> Calibrated/1
  Relative Encoder/1 -> Encoder Initializer/2, Unwrapper/1
  Unwrapper/1 -> Encoder Initializer/1
  Absolute Encoder/1 -> Encoder Initializer/3

== system HardwareIO/Hardware I//O/Input/Handwheel Scaling & Initialization/Handwheel Sensor Fault Detection ==
  Relative : Inport
  Absolute : Inport  Port=2
  Descision Logic : Subsystem
  Enable Timer : Subsystem
  Fault Detection1 : Subsystem
  Ground : Ground
  Switch Over : Subsystem
  Terminator : Terminator
  Primary : Outport
  Secondary : Outport  Port=2
  Fault : Outport  Port=3
  wires:
  Ground/1 -> Switch Over/2(Chooser)
  Fault Detection1/3(Frozen) -> Descision Logic/3(Frozen)
  Fault Detection1/4(Partially Frozen) -> Descision Logic/4(Partially Frozen)
  Enable Timer/1(Enable) -> Descision Logic/5(Enable)
  Switch Over/2(Secondary) -> Secondary/1
  Descision Logic/2(Fault) -> Fault/1
  Switch Over/1(Primary) -> Primary/1
  Descision Logic/1(Best Bet) -> Terminator/1
  Fault Detection1/1(Disparity) -> Descision Logic/1(Disparity)
  Absolute/1 -> Fault Detection1/2(Absolute), Switch Over/3(Absolute)
  Fault Detection1/2(Jump) -> Descision Logic/2(Jump)
  Relative/1 -> Fault Detection1/1(Relative), Switch Over/1(Relative)

== system HardwareIO/Hardware I//O/Input/Rear Wheel Speed Processing/Speed Calc ==
  Distance : Inport
  Clock : Clock
  Difference : DiscreteTransferFcn  Numerator=[1 -1]  Denominator=[1 0]
  Mux : Mux  Inputs=2
  Unwrapping : Fcn  Expr=((u<=-range/2) - (u>=range/2)) * range + u
  Zero @ t=0; normal otherwise : Fcn  Expr=(u(2)>0) * u(1)
  Speed : Outport
  wires:
  Unwrapping/1 -> Mux/1
  Distance/1 -> Difference/1
  Difference/1 -> Unwrapping/1
  Clock/1 -> Mux/2
  Mux/1 -> Zero @ t=0; normal otherwise/1
  Zero @ t=0; normal otherwise/1 -> Speed/1

== system HardwareIO/Hardware I//O/Input/Rear Wheel Speed Processing/Speed Calc1 ==
  Distance : Inport
  Clock : Clock
  Difference : DiscreteTransferFcn  Numerator=[1 -1]  Denominator=[1 0]
  Mux : Mux  Inputs=2
  Unwrapping : Fcn  Expr=((u<=-range/2) - (u>=range/2)) * range + u
  Zero @ t=0; normal otherwise : Fcn  Expr=(u(2)>0) * u(1)
  Speed : Outport
  wires:
  Zero @ t=0; normal otherwise/1 -> Speed/1
  Mux/1 -> Zero @ t=0; normal otherwise/1
  Clock/1 -> Mux/2
  Difference/1 -> Unwrapping/1
  Distance/1 -> Difference/1
  Unwrapping/1 -> Mux/1

== system HardwareIO/Hardware I//O/Input/Steering Motor Encoder Initialization/Left ==
  Encoder : Inport
  Potentiometer : Inport  Port=2
  Encoder Initializer : S-Function  FunctionName=encoderinit  Parameters=sampleTime,firstDelay,secondDelay  EnableBusSupport=off  mask{sampleTime=Ts, firstDelay=.1, secondDelay=.2}
      mask prompts: sampleTime "Sample time"; firstDelay "First calibration time"; secondDelay "Second calibration time"
      mask Display:
      | port_label('input',1,'Unwrapped');
      | port_label('input',2,'Raw');
      | port_label('input',3,'Pot');
      | port_label('output',1,'Calibrated');
  Unwrapper : S-Function  FunctionName=unwrapper  Parameters=Ts,2*pi  EnableBusSupport=off
      mask Display: disp('2*pi')
  Calibrated : Outport
  wires:
  Potentiometer/1 -> Encoder Initializer/3
  Unwrapper/1 -> Encoder Initializer/1
  Encoder/1 -> Unwrapper/1, Encoder Initializer/2
  Encoder Initializer/1 -> Calibrated/1

== system HardwareIO/Hardware I//O/Input/Steering Motor Encoder Initialization/Right ==
  Encoder : Inport
  Potentiometer : Inport  Port=2
  Encoder Initializer : S-Function  FunctionName=encoderinit  Parameters=sampleTime,firstDelay,secondDelay  EnableBusSupport=off  mask{sampleTime=Ts, firstDelay=.1, secondDelay=.2}
      mask prompts: sampleTime "Sample time"; firstDelay "First calibration time"; secondDelay "Second calibration time"
      mask Display:
      | port_label('input',1,'Unwrapped');
      | port_label('input',2,'Raw');
      | port_label('input',3,'Pot');
      | port_label('output',1,'Calibrated');
  Unwrapper : S-Function  FunctionName=unwrapper  Parameters=Ts,2*pi  EnableBusSupport=off
      mask Display: disp('2*pi')
  Calibrated : Outport
  wires:
  Encoder/1 -> Unwrapper/1, Encoder Initializer/2
  Unwrapper/1 -> Encoder Initializer/1
  Encoder Initializer/1 -> Calibrated/1
  Potentiometer/1 -> Encoder Initializer/3

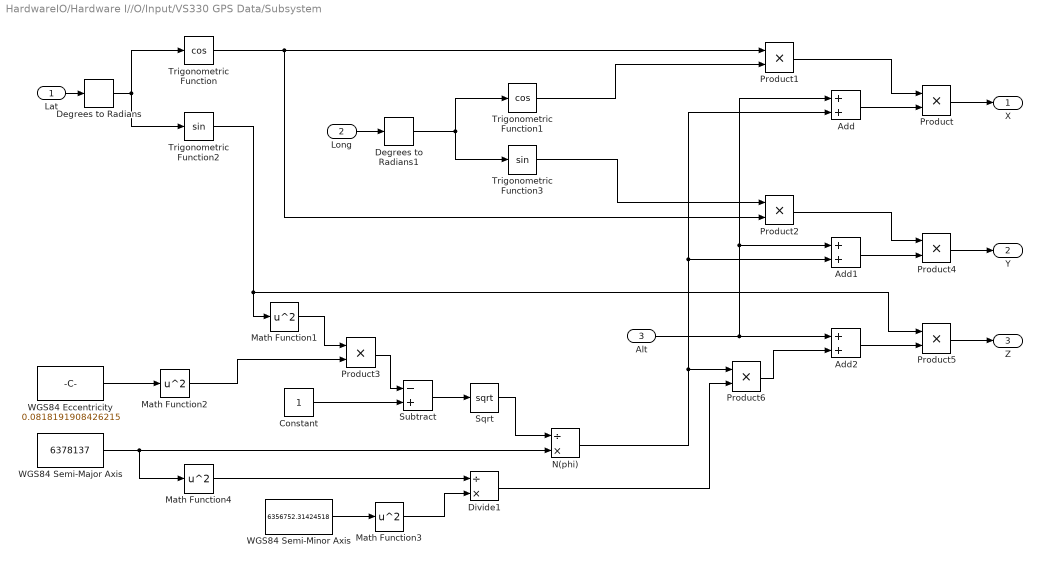
== system HardwareIO/Hardware I//O/Input/VS330 GPS Data/Subsystem ==
  Lat : Inport
  Long : Inport  Port=2
  Alt : Inport  Port=3
  Add : Sum
  Add1 : Sum
  Add2 : Sum
  Constant : Constant
  Degrees to Radians : simulink_extras/Transformations/Degrees to Radians
  Degrees to Radians1 : simulink_extras/Transformations/Degrees to Radians
  Divide1 : Product  Inputs=/*
  Math Function{1..4} (4 alike) : Math  Operator=square  SaturateOnIntegerOverflow=on
  N(phi) : Product  Inputs=/*
  Product{,1..6} (7 alike) : Product
  Sqrt : Sqrt  SaturateOnIntegerOverflow=on
  Subtract : Sum  Inputs=-+
  Trigonometric Function : Trigonometry  Operator=cos
  Trigonometric Function1 : Trigonometry  Operator=cos
  Trigonometric Function2 : Trigonometry
  Trigonometric Function3 : Trigonometry
  WGS84 Eccentricity : Constant  Value=0.0818191908426215
  WGS84 Semi-Major Axis : Constant  Value=6378137
  WGS84 Semi-Minor Axis : Constant  Value=6356752.31424518
  X : Outport
  Y : Outport  Port=2
  Z : Outport  Port=3
  wires:
  Degrees to Radians1/1 -> Trigonometric Function1/1, Trigonometric Function3/1
  Degrees to Radians/1 -> Trigonometric Function2/1, Trigonometric Function/1
  Trigonometric Function3/1 -> Product2/1
  Math Function4/1 -> Divide1/1
  Math Function3/1 -> Divide1/2
  Divide1/1 -> Product6/2
  Product6/1 -> Add2/2
  N(phi)/1 -> Add1/2, Add/2, Product6/1
  WGS84 Semi-Minor Axis/1 -> Math Function3/1
  WGS84 Semi-Major Axis/1 -> N(phi)/2, Math Function4/1
  Product3/1 -> Subtract/1
  Sqrt/1 -> N(phi)/1
  Constant/1 -> Subtract/2
  Math Function1/1 -> Product3/1
  Math Function2/1 -> Product3/2
  Subtract/1 -> Sqrt/1
  Trigonometric Function2/1 -> Product5/1, Math Function1/1
  Trigonometric Function1/1 -> Product1/2
  Trigonometric Function/1 -> Product1/1, Product2/2
  Add2/1 -> Product5/2
  Add1/1 -> Product4/2
  Product2/1 -> Product4/1
  Product1/1 -> Product/1
  Product/1 -> X/1
  Product4/1 -> Y/1
  Product5/1 -> Z/1
  Add/1 -> Product/2
  Alt/1 -> Add2/1, Add1/1, Add/1
  Long/1 -> Degrees to Radians1/1
  Lat/1 -> Degrees to Radians/1
  WGS84 Eccentricity/1 -> Math Function2/1

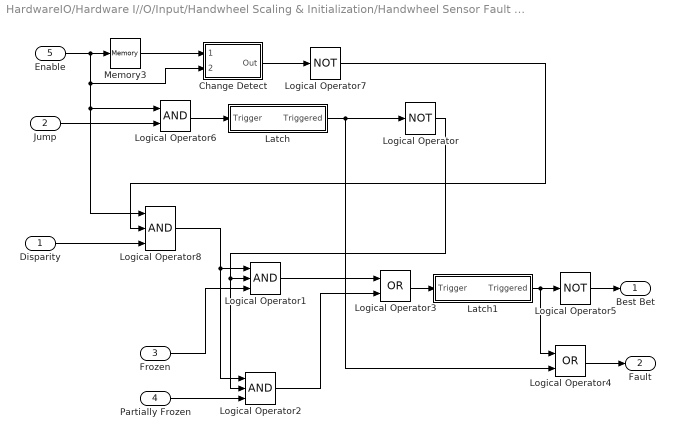
== system HardwareIO/Hardware I//O/Input/Handwheel Scaling & Initialization/Handwheel Sensor Fault Detection/Descision Logic ==
  Disparity : Inport
  Jump : Inport  Port=2
  Frozen : Inport  Port=3
  Partially Frozen : Inport  Port=4
  Enable : Inport  Port=5
  Change Detect : Subsystem
  Latch : Subsystem
  Latch1 : Subsystem
  Logical Operator : Logic  Operator=NOT  AllPortsSameDT=off  OutDataTypeStr=float('double')
  Logical Operator1 : Logic  Inputs=3  AllPortsSameDT=off  OutDataTypeStr=float('double')
  Logical Operator2 : Logic  Inputs=3  AllPortsSameDT=off  OutDataTypeStr=float('double')
  Logical Operator3 : Logic  Operator=OR  AllPortsSameDT=off  OutDataTypeStr=float('double')
  Logical Operator4 : Logic  Operator=OR  AllPortsSameDT=off  OutDataTypeStr=float('double')
  Logical Operator5 : Logic  Operator=NOT  AllPortsSameDT=off  OutDataTypeStr=float('double')
  Logical Operator6 : Logic  AllPortsSameDT=off  OutDataTypeStr=float('double')
  Logical Operator7 : Logic  Operator=NOT  AllPortsSameDT=off  OutDataTypeStr=float('double')
  Logical Operator8 : Logic  Inputs=3  AllPortsSameDT=off  OutDataTypeStr=float('double')
  Memory3 : Memory  InheritSampleTime=on
  Best Bet : Outport
  Fault : Outport  Port=2
  wires:
  Logical Operator6/1 -> Latch/1(Trigger)
  Disparity/1 -> Logical Operator8/3
  Logical Operator7/1 -> Logical Operator8/2
  Logical Operator8/1 -> Logical Operator2/1, Logical Operator1/1
  Change Detect/1(Out) -> Logical Operator7/1
  Jump/1 -> Logical Operator6/2
  Memory3/1 -> Change Detect/1(1)
  Enable/1 -> Logical Operator8/1, Logical Operator6/1, Change Detect/2(2), Memory3/1
  Logical Operator5/1 -> Best Bet/1
  Logical Operator4/1 -> Fault/1
  Logical Operator/1 -> Logical Operator2/2, Logical Operator1/2
  Latch/1(Triggered) -> Logical Operator4/2, Logical Operator/1
  Logical Operator2/1 -> Logical Operator3/2
  Logical Operator1/1 -> Logical Operator3/1
  Logical Operator3/1 -> Latch1/1(Trigger)
  Partially Frozen/1 -> Logical Operator2/3
  Frozen/1 -> Logical Operator1/3
  Latch1/1(Triggered) -> Logical Operator5/1, Logical Operator4/1

== system HardwareIO/Hardware I//O/Input/Handwheel Scaling & Initialization/Handwheel Sensor Fault Detection/Enable Timer ==
  Clock : Clock
  Constant : Constant
  Relational Operator : RelationalOperator  Operator=>  OutDataTypeStr=float('double')
  Enable : Outport
  wires:
  Relational Operator/1 -> Enable/1
  Constant/1 -> Relational Operator/2
  Clock/1 -> Relational Operator/1

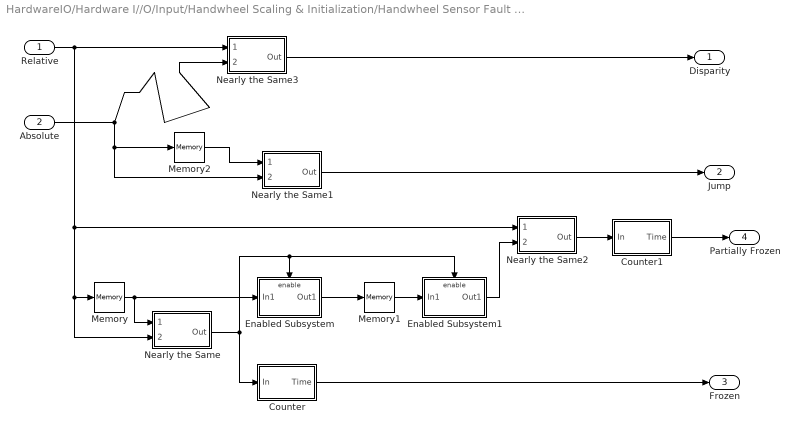
== system HardwareIO/Hardware I//O/Input/Handwheel Scaling & Initialization/Handwheel Sensor Fault Detection/Fault Detection1 ==
  Relative : Inport
  Absolute : Inport  Port=2
  Counter : Subsystem
  Counter1 : Subsystem
  Enabled Subsystem : Subsystem  TreatAsAtomicUnit=on
  Enabled Subsystem1 : Subsystem  TreatAsAtomicUnit=on
  Memory : Memory  InheritSampleTime=on
  Memory1 : Memory  InheritSampleTime=on
  Memory2 : Memory  InheritSampleTime=on
  Nearly the Same : Subsystem
  Nearly the Same1 : Subsystem
  Nearly the Same2 : Subsystem
  Nearly the Same3 : Subsystem
  Disparity : Outport
  Jump : Outport  Port=2
  Frozen : Outport  Port=3
  Partially Frozen : Outport  Port=4
  wires:
  Nearly the Same1/1(Out) -> Jump/1
  Memory2/1 -> Nearly the Same1/1(1)
  Counter1/1(Time) -> Partially Frozen/1
  Nearly the Same2/1(Out) -> Counter1/1(In)
  Nearly the Same/1(Out) -> Enabled Subsystem/Enable, Enabled Subsystem1/Enable, Counter/1(In)
  Counter/1(Time) -> Frozen/1
  Memory1/1 -> Enabled Subsystem1/1(In1)
  Enabled Subsystem1/1(Out1) -> Nearly the Same2/2(2)
  Enabled Subsystem/1(Out1) -> Memory1/1
  Memory/1 -> Nearly the Same/1(1), Enabled Subsystem/1(In1)
  Nearly the Same3/1(Out) -> Disparity/1
  Absolute/1 -> Nearly the Same1/2(2), Memory2/1, Nearly the Same3/2(2)
  Relative/1 -> Memory/1, Nearly the Same/2(2), Nearly the Same2/1(1), Nearly the Same3/1(1)

== system HardwareIO/Hardware I//O/Input/Handwheel Scaling & Initialization/Handwheel Sensor Fault Detection/Switch Over ==
  Relative : Inport
  Chooser : Inport  Port=2
  Absolute : Inport  Port=3
  Logical Operator5 : Logic  Operator=NOT  AllPortsSameDT=off  OutDataTypeStr=float('double')
  Switch : Switch  Threshold=.5
  Switch1 : Switch  Threshold=.5
  Primary : Outport
  Secondary : Outport  Port=2
  wires:
  Chooser/1 -> Switch/2, Logical Operator5/1
  Switch1/1 -> Primary/1
  Absolute/1 -> Switch1/3, Switch/3
  Relative/1 -> Switch1/1, Switch/1
  Logical Operator5/1 -> Switch1/2
  Switch/1 -> Secondary/1

== system HardwareIO/Hardware I//O/Input/Handwheel Scaling & Initialization/Handwheel Sensor Fault Detection/Descision Logic/Change Detect ==
  1 : Inport
  2 : Inport  Port=2
  Abs : Abs
  Constant : Constant  Value=.1
  Relational Operator : RelationalOperator  Operator=>  OutDataTypeStr=float('double')
  Sum2 : Sum  Inputs=|+-
  Out : Outport
  wires:
  Constant/1 -> Relational Operator/2
  Relational Operator/1 -> Out/1
  2/1 -> Sum2/2
  Abs/1 -> Relational Operator/1
  1/1 -> Sum2/1
  Sum2/1 -> Abs/1

== system HardwareIO/Hardware I//O/Input/Handwheel Scaling & Initialization/Handwheel Sensor Fault Detection/Descision Logic/Latch ==
  Trigger : Inport
  Constant : Constant
  Enabled Subsystem : Subsystem  TreatAsAtomicUnit=on
  Triggered : Outport
  wires:
  Constant/1 -> Enabled Subsystem/1(In1)
  Enabled Subsystem/1(Out1) -> Triggered/1
  Trigger/1 -> Enabled Subsystem/Enable

== system HardwareIO/Hardware I//O/Input/Handwheel Scaling & Initialization/Handwheel Sensor Fault Detection/Descision Logic/Latch1 ==
  Trigger : Inport
  Constant : Constant
  Enabled Subsystem : Subsystem  TreatAsAtomicUnit=on
  Triggered : Outport
  wires:
  Constant/1 -> Enabled Subsystem/1(In1)
  Enabled Subsystem/1(Out1) -> Triggered/1
  Trigger/1 -> Enabled Subsystem/Enable

== system HardwareIO/Hardware I//O/Input/Handwheel Scaling & Initialization/Handwheel Sensor Fault Detection/Fault Detection1/Counter ==
  In : Inport
  Constant : Constant  Value=10
  Constant1 : Constant
  Discrete-Time Integrator : DiscreteIntegrator  ExternalReset=level  SampleTime=-1  LimitOutput=on  UpperSaturationLimit=10  LowerSaturationLimit=-10  ICPrevOutput=DiscIntNeverNeededParam  ICPrevScaledInput=DiscIntNeverNeededParam
  Relational Operator2 : RelationalOperator  Operator=>  OutDataTypeStr=float('double')
  Time : Outport
  wires:
  In/1 -> Discrete-Time Integrator/2
  Constant/1 -> Discrete-Time Integrator/1
  Discrete-Time Integrator/1 -> Relational Operator2/1
  Constant1/1 -> Relational Operator2/2
  Relational Operator2/1 -> Time/1

== system HardwareIO/Hardware I//O/Input/Handwheel Scaling & Initialization/Handwheel Sensor Fault Detection/Fault Detection1/Counter1 ==
  In : Inport
  Constant : Constant  Value=10
  Constant1 : Constant
  Discrete-Time Integrator : DiscreteIntegrator  ExternalReset=level  SampleTime=-1  LimitOutput=on  UpperSaturationLimit=10  LowerSaturationLimit=-10  ICPrevOutput=DiscIntNeverNeededParam  ICPrevScaledInput=DiscIntNeverNeededParam
  Relational Operator2 : RelationalOperator  Operator=>  OutDataTypeStr=float('double')
  Time : Outport
  wires:
  In/1 -> Discrete-Time Integrator/2
  Constant/1 -> Discrete-Time Integrator/1
  Discrete-Time Integrator/1 -> Relational Operator2/1
  Constant1/1 -> Relational Operator2/2
  Relational Operator2/1 -> Time/1

== system HardwareIO/Hardware I//O/Input/Handwheel Scaling & Initialization/Handwheel Sensor Fault Detection/Fault Detection1/Enabled Subsystem ==
  In1 : Inport
  Enable : EnablePort
  Out1 : Outport
  wires:
  In1/1 -> Out1/1

== system HardwareIO/Hardware I//O/Input/Handwheel Scaling & Initialization/Handwheel Sensor Fault Detection/Fault Detection1/Enabled Subsystem1 ==
  In1 : Inport
  Enable : EnablePort
  Out1 : Outport
  wires:
  In1/1 -> Out1/1

== system HardwareIO/Hardware I//O/Input/Handwheel Scaling & Initialization/Handwheel Sensor Fault Detection/Fault Detection1/Nearly the Same ==
  1 : Inport
  2 : Inport  Port=2
  Abs : Abs
  Constant : Constant  Value=.0001
  Relational Operator : RelationalOperator  Operator=>  OutDataTypeStr=float('double')
  Sum2 : Sum  Inputs=|+-
  Out : Outport
  wires:
  Sum2/1 -> Abs/1
  1/1 -> Sum2/1
  Abs/1 -> Relational Operator/1
  2/1 -> Sum2/2
  Relational Operator/1 -> Out/1
  Constant/1 -> Relational Operator/2

== system HardwareIO/Hardware I//O/Input/Handwheel Scaling & Initialization/Handwheel Sensor Fault Detection/Fault Detection1/Nearly the Same1 ==
  1 : Inport
  2 : Inport  Port=2
  Abs : Abs
  Constant : Constant  Value=.1
  Relational Operator : RelationalOperator  Operator=>  OutDataTypeStr=float('double')
  Sum2 : Sum  Inputs=|+-
  Out : Outport
  wires:
  Sum2/1 -> Abs/1
  1/1 -> Sum2/1
  Abs/1 -> Relational Operator/1
  2/1 -> Sum2/2
  Relational Operator/1 -> Out/1
  Constant/1 -> Relational Operator/2

== system HardwareIO/Hardware I//O/Input/Handwheel Scaling & Initialization/Handwheel Sensor Fault Detection/Fault Detection1/Nearly the Same2 ==
  1 : Inport
  2 : Inport  Port=2
  Abs : Abs
  Constant : Constant  Value=.0001
  Relational Operator : RelationalOperator  Operator=>  OutDataTypeStr=float('double')
  Sum2 : Sum  Inputs=|+-
  Out : Outport
  wires:
  Constant/1 -> Relational Operator/2
  Relational Operator/1 -> Out/1
  2/1 -> Sum2/2
  Abs/1 -> Relational Operator/1
  1/1 -> Sum2/1
  Sum2/1 -> Abs/1

== system HardwareIO/Hardware I//O/Input/Handwheel Scaling & Initialization/Handwheel Sensor Fault Detection/Fault Detection1/Nearly the Same3 ==
  1 : Inport
  2 : Inport  Port=2
  Abs : Abs
  Constant : Constant  Value=.2
  Relational Operator : RelationalOperator  Operator=>  OutDataTypeStr=float('double')
  Sum2 : Sum  Inputs=|+-
  Out : Outport
  wires:
  Constant/1 -> Relational Operator/2
  Relational Operator/1 -> Out/1
  2/1 -> Sum2/2
  Abs/1 -> Relational Operator/1
  1/1 -> Sum2/1
  Sum2/1 -> Abs/1

== system HardwareIO/Hardware I//O/Input/Handwheel Scaling & Initialization/Handwheel Sensor Fault Detection/Descision Logic/Latch/Enabled Subsystem ==
  In1 : Inport
  Enable : EnablePort
  Out1 : Outport
  wires:
  In1/1 -> Out1/1

== system HardwareIO/Hardware I//O/Input/Handwheel Scaling & Initialization/Handwheel Sensor Fault Detection/Descision Logic/Latch1/Enabled Subsystem ==
  In1 : Inport
  Enable : EnablePort
  Out1 : Outport
  wires:
  In1/1 -> Out1/1
